simulink model "VehDyn14DOF"  (R2024b)
settings: Solver=VariableStepAuto  StartTime=0.0  StopTime=inf  FixedStep=0.001  RelTol=1e-3
model workspace (MAT data in the model file):
  ssEnable : Simulink.Parameter (value not decoded)
  xdot_r : Simulink.Parameter (value not decoded)
values from neighbouring files (symbols this model uses):
  AccPwrbp = 0.0 3.0779560993538198    [vehDyn14DOF.sldd]
  AccSpdbp = 256.49641719585139 641.24104298962845    [vehDyn14DOF.sldd]
  Downshift_Speeds = 9.5625 12.9375 16.3125 19.6875 23.0625 26.4375 29.8125 33.1875 36.5625 39.9375 43.3125 46.687499999999986 47.8125 51.187499999999986 54.562499999999986 57.9375 59.0625 62.4375 65.8125 69.1875 68.90625 72.84375 76.78125 80.71875 78.75 83.25 87.75 92.25    [vehDyn14DOF.sldd]
  egoVehDyn = egoVehicleDynamicsParamsFromRR(egoInitialPose, actorProfiles(egoActorID))    [helperSLTrajectoryFollowerWithRRScenarioSetup.m]
  EngRevLim = 7000.0    [vehDyn14DOF.sldd]
  F0z = 2886.0 2907.0    [vehDyn14DOF.sldd]
  Iz = evalin('base','Iz')    [helperSLTrajectoryFollowerWithRRScenarioSetup.m]
  lf = evalin('base','lf')    [helperSLTrajectoryFollowerWithRRScenarioSetup.m]
  lr = evalin('base','lr')    [helperSLTrajectoryFollowerWithRRScenarioSetup.m]
  m = worldActors(idx).actor_runtime.pose.matrix    [helperSLTrajectoryFollowerWithRRScenarioSetup.m]
  Pedal_Positions = 0.1 0.4 0.5 0.9    [vehDyn14DOF.sldd]
  steerGear = evalin('base', 'steerGear')    [helperSLTrajectoryFollowerWithRRScenarioSetup.m]
  steeringGain = evalin('base', 'steeringGain')    [helperSLTrajectoryFollowerWithRRScenarioSetup.m]
  steerLimit = evalin('base', 'steerLimit')    [helperSLTrajectoryFollowerWithRRScenarioSetup.m]
  Trans = 0.01    [vehDyn14DOF.sldd]
  Upshift_Speeds = 12.9375 16.3125 19.6875 33.0 26.4375 29.8125 33.1875 52.5 39.9375 43.3125 46.687499999999986 77.25 51.187499999999986 54.562499999999986 57.9375 100.5 62.4375 65.8125 69.1875 138.75 72.84375 76.78125 80.71875 161.875 83.25 87.75 92.25 185.0    [vehDyn14DOF.sldd]
  VEH = 1575.0    [vehDyn14DOF.sldd]
symbols that are objects in the model workspace (value not decoded): ssEnable, xdot_r
undefined symbols (not defined in the file or in its folder): AccelCmd, CurvGradRef, CurvRef, DecelCmd, DiscIntNeverNeededParam, EnblAccelCmd, EnblDecelCmd, EnblSteerCmd, GearCmd, Gnd, lambda_mux, lambda_muy, LngRef, LtrRef, max_ac, max_dc, PhiRef, SteerCmd, SteerZero, Wind, XRef, YRef, Z
libraries: simulink x14, autolibutils x13, autolibsharedcoupling x11, vehdynlibtire x10, vehdynlibsuspension x8, sharedtransform x5, autolibshareddiff x5, shared6dof x2, slpidlib x1, autolibtranscontrolscommon x1, vehdynlibdriver x1, autolibshared x1
(part 10 of 10)

== system VehDyn14DOF/Passenger Vehicle/Chassis and Tires/Wheels and Tires/VDBS/Tires/MF Tires/Fy ==
  In1 : Inport
  In2 : Inport  Port=2
  In3 : Inport  Port=3
  In4 : Inport  Port=4
  Bus Selector{,1..3} (4 alike) : BusSelector  OutputSignals=Fy
  Vector Concatenate : Concatenate  NumInputs=4
  Out1 : Outport  VectorParamsAs1DForOutWhenUnconnected=off
  wires:
  Vector Concatenate/1 -> Out1/1
  In1/1 -> Bus Selector/1
  Bus Selector/1 -> Vector Concatenate/1  "<Fy>"
  In2/1 -> Bus Selector1/1
  In3/1 -> Bus Selector2/1
  In4/1 -> Bus Selector3/1
  Bus Selector1/1 -> Vector Concatenate/2  "<Fy>"
  Bus Selector2/1 -> Vector Concatenate/3  "<Fy>"
  Bus Selector3/1 -> Vector Concatenate/4  "<Fy>"

== system VehDyn14DOF/Passenger Vehicle/Chassis and Tires/Wheels and Tires/VDBS/Tires/MF Tires/Fz ==
  In1 : Inport
  In2 : Inport  Port=2
  In3 : Inport  Port=3
  In4 : Inport  Port=4
  Bus Selector{,1..3} (4 alike) : BusSelector  OutputSignals=Fz
  Vector Concatenate : Concatenate  NumInputs=4
  Out1 : Outport  VectorParamsAs1DForOutWhenUnconnected=off
  wires:
  Vector Concatenate/1 -> Out1/1
  In1/1 -> Bus Selector/1
  Bus Selector/1 -> Vector Concatenate/1  "<Fz>"
  In2/1 -> Bus Selector1/1
  In3/1 -> Bus Selector2/1
  In4/1 -> Bus Selector3/1
  Bus Selector1/1 -> Vector Concatenate/2  "<Fz>"
  Bus Selector2/1 -> Vector Concatenate/3  "<Fz>"
  Bus Selector3/1 -> Vector Concatenate/4  "<Fz>"

== system VehDyn14DOF/Passenger Vehicle/Chassis and Tires/Wheels and Tires/VDBS/Tires/MF Tires/Mx ==
  In1 : Inport
  In2 : Inport  Port=2
  In3 : Inport  Port=3
  In4 : Inport  Port=4
  Bus Selector{,1..3} (4 alike) : BusSelector  OutputSignals=Mx
  Vector Concatenate : Concatenate  NumInputs=4
  Out1 : Outport  VectorParamsAs1DForOutWhenUnconnected=off
  wires:
  Vector Concatenate/1 -> Out1/1
  In1/1 -> Bus Selector/1
  Bus Selector/1 -> Vector Concatenate/1  "<Mx>"
  In2/1 -> Bus Selector1/1
  In3/1 -> Bus Selector2/1
  In4/1 -> Bus Selector3/1
  Bus Selector1/1 -> Vector Concatenate/2  "<Mx>"
  Bus Selector2/1 -> Vector Concatenate/3  "<Mx>"
  Bus Selector3/1 -> Vector Concatenate/4  "<Mx>"

== system VehDyn14DOF/Passenger Vehicle/Chassis and Tires/Wheels and Tires/VDBS/Tires/MF Tires/My ==
  In1 : Inport
  In2 : Inport  Port=2
  In3 : Inport  Port=3
  In4 : Inport  Port=4
  Bus Selector{,1..3} (4 alike) : BusSelector  OutputSignals=My
  Vector Concatenate : Concatenate  NumInputs=4
  Out1 : Outport  VectorParamsAs1DForOutWhenUnconnected=off
  wires:
  Bus Selector3/1 -> Vector Concatenate/4  "<My>"
  Bus Selector2/1 -> Vector Concatenate/3  "<My>"
  Bus Selector1/1 -> Vector Concatenate/2  "<My>"
  In4/1 -> Bus Selector3/1
  In3/1 -> Bus Selector2/1
  In2/1 -> Bus Selector1/1
  Bus Selector/1 -> Vector Concatenate/1  "<My>"
  In1/1 -> Bus Selector/1
  Vector Concatenate/1 -> Out1/1

== system VehDyn14DOF/Passenger Vehicle/Chassis and Tires/Wheels and Tires/VDBS/Tires/MF Tires/Mz ==
  In1 : Inport
  In2 : Inport  Port=2
  In3 : Inport  Port=3
  In4 : Inport  Port=4
  Bus Selector{,1..3} (4 alike) : BusSelector  OutputSignals=Mz
  Vector Concatenate : Concatenate  NumInputs=4
  Out1 : Outport  VectorParamsAs1DForOutWhenUnconnected=off
  wires:
  Bus Selector3/1 -> Vector Concatenate/4  "<Mz>"
  Bus Selector2/1 -> Vector Concatenate/3  "<Mz>"
  Bus Selector1/1 -> Vector Concatenate/2  "<Mz>"
  In4/1 -> Bus Selector3/1
  In3/1 -> Bus Selector2/1
  In2/1 -> Bus Selector1/1
  Bus Selector/1 -> Vector Concatenate/1  "<Mz>"
  In1/1 -> Bus Selector/1
  Vector Concatenate/1 -> Out1/1

== system VehDyn14DOF/Passenger Vehicle/Chassis and Tires/Wheels and Tires/VDBS/Tires/MF Tires/Re ==
  In1 : Inport
  In2 : Inport  Port=2
  In3 : Inport  Port=3
  In4 : Inport  Port=4
  Bus Selector{,1..3} (4 alike) : BusSelector  OutputSignals=Re
  Vector Concatenate : Concatenate  NumInputs=4
  Out1 : Outport  VectorParamsAs1DForOutWhenUnconnected=off
  wires:
  Vector Concatenate/1 -> Out1/1
  In1/1 -> Bus Selector/1
  Bus Selector/1 -> Vector Concatenate/1  "<Re>"
  In2/1 -> Bus Selector1/1
  In3/1 -> Bus Selector2/1
  In4/1 -> Bus Selector3/1
  Bus Selector1/1 -> Vector Concatenate/2  "<Re>"
  Bus Selector2/1 -> Vector Concatenate/3  "<Re>"
  Bus Selector3/1 -> Vector Concatenate/4  "<Re>"

== system VehDyn14DOF/Passenger Vehicle/Chassis and Tires/Wheels and Tires/VDBS/Tires/MF Tires/alpha ==
  In1 : Inport
  In2 : Inport  Port=2
  In3 : Inport  Port=3
  In4 : Inport  Port=4
  Bus Selector{,1..3} (4 alike) : BusSelector  OutputSignals=Alpha
  Vector Concatenate : Concatenate  NumInputs=4
  Out1 : Outport  VectorParamsAs1DForOutWhenUnconnected=off
  wires:
  Vector Concatenate/1 -> Out1/1
  In1/1 -> Bus Selector/1
  Bus Selector/1 -> Vector Concatenate/1  "<Alpha>"
  In2/1 -> Bus Selector1/1
  In3/1 -> Bus Selector2/1
  In4/1 -> Bus Selector3/1
  Bus Selector1/1 -> Vector Concatenate/2  "<Alpha>"
  Bus Selector2/1 -> Vector Concatenate/3  "<Alpha>"
  Bus Selector3/1 -> Vector Concatenate/4  "<Alpha>"

== system VehDyn14DOF/Passenger Vehicle/Chassis and Tires/Wheels and Tires/VDBS/Tires/MF Tires/kappa ==
  In1 : Inport
  In2 : Inport  Port=2
  In3 : Inport  Port=3
  In4 : Inport  Port=4
  Bus Selector{,1..3} (4 alike) : BusSelector  OutputSignals=Kappa
  Vector Concatenate : Concatenate  NumInputs=4
  Out1 : Outport  VectorParamsAs1DForOutWhenUnconnected=off
  wires:
  Bus Selector3/1 -> Vector Concatenate/4  "<Kappa>"
  Bus Selector2/1 -> Vector Concatenate/3  "<Kappa>"
  Bus Selector1/1 -> Vector Concatenate/2  "<Kappa>"
  In4/1 -> Bus Selector3/1
  In3/1 -> Bus Selector2/1
  In2/1 -> Bus Selector1/1
  Bus Selector/1 -> Vector Concatenate/1  "<Kappa>"
  In1/1 -> Bus Selector/1
  Vector Concatenate/1 -> Out1/1

== system VehDyn14DOF/Passenger Vehicle/Chassis and Tires/Wheels and Tires/VDBS/Tires/MF Tires/omega ==
  In1 : Inport
  In2 : Inport  Port=2
  In3 : Inport  Port=3
  In4 : Inport  Port=4
  Bus Selector{,1..3} (4 alike) : BusSelector  OutputSignals=Omega
  Vector Concatenate : Concatenate  NumInputs=4
  Out1 : Outport  VectorParamsAs1DForOutWhenUnconnected=off
  wires:
  In1/1 -> Bus Selector/1
  Bus Selector/1 -> Vector Concatenate/1  "<Omega>"
  In2/1 -> Bus Selector1/1
  In3/1 -> Bus Selector2/1
  In4/1 -> Bus Selector3/1
  Bus Selector1/1 -> Vector Concatenate/2  "<Omega>"
  Bus Selector2/1 -> Vector Concatenate/3  "<Omega>"
  Bus Selector3/1 -> Vector Concatenate/4  "<Omega>"
  Vector Concatenate/1 -> Out1/1

== system VehDyn14DOF/Passenger Vehicle/Chassis and Tires/Wheels and Tires/VDBS/Tires/MF Tires/z ==
  In1 : Inport
  In2 : Inport  Port=2
  In3 : Inport  Port=3
  In4 : Inport  Port=4
  Bus Selector{,1..3} (4 alike) : BusSelector  OutputSignals=z
  Vector Concatenate : Concatenate  NumInputs=4
  Out1 : Outport  VectorParamsAs1DForOutWhenUnconnected=off
  wires:
  Bus Selector3/1 -> Vector Concatenate/4  "<z>"
  Bus Selector2/1 -> Vector Concatenate/3  "<z>"
  Bus Selector1/1 -> Vector Concatenate/2  "<z>"
  In4/1 -> Bus Selector3/1
  In3/1 -> Bus Selector2/1
  In2/1 -> Bus Selector1/1
  Bus Selector/1 -> Vector Concatenate/1  "<z>"
  In1/1 -> Bus Selector/1
  Vector Concatenate/1 -> Out1/1

== system VehDyn14DOF/Passenger Vehicle/Chassis and Tires/Wheels and Tires/VDBS/Tires/MF Tires/zdot ==
  In1 : Inport
  In2 : Inport  Port=2
  In3 : Inport  Port=3
  In4 : Inport  Port=4
  Bus Selector{,1..3} (4 alike) : BusSelector  OutputSignals=zdot
  Vector Concatenate : Concatenate  NumInputs=4
  Out1 : Outport  VectorParamsAs1DForOutWhenUnconnected=off
  wires:
  Vector Concatenate/1 -> Out1/1
  In1/1 -> Bus Selector/1
  Bus Selector/1 -> Vector Concatenate/1  "<zdot>"
  In2/1 -> Bus Selector1/1
  In3/1 -> Bus Selector2/1
  In4/1 -> Bus Selector3/1
  Bus Selector1/1 -> Vector Concatenate/2  "<zdot>"
  Bus Selector2/1 -> Vector Concatenate/3  "<zdot>"
  Bus Selector3/1 -> Vector Concatenate/4  "<zdot>"

== stateflow chart VehDyn14DOF/Controllers/Transmission Controller/Transmission Controller/TCM/TCM Shift Controller ==
  settings: sampleTime=0.01
  state GearCmd [parallel]
    settings: executionOrder=1
    state Neutral
      en:
      GearCmd = 0;
    state G1
      en:
      GearCmd = 1;
    state G2
      en:
      GearCmd = 2;
      du:
      [SpdThr] = calc(2,pedal,speed);
    state G3
      en:
      GearCmd = 3;
      du:
      [SpdThr] = calc(3,pedal,speed);
    state G8
      en:
      GearCmd = 8;
    state G7
      en:
      GearCmd = 7;
    state G6
      en:
      GearCmd = 6;
    state G5
      en:GearCmd=5;
      du:[SpdThr]=calc(5,pedal,speed);
    state G4
      en:
      GearCmd = 4;
      du:
      [SpdThr] = calc(4,pedal,speed);
    (default) -> Neutral
    Neutral -> G1 : [~Neutral]
    G1 -> G2 [order 1] : Up
    G2 -> G3 [order 1] : Up
    G1 -> Neutral [order 2] : [Neutral]
    G2 -> G1 [order 2] : Down
    G3 -> G2 [order 2] : Down
    G3 -> G4 [order 1] : Up
    G4 -> G3 [order 2] : Down
    G7 -> G8 [order 1] : Up
    G5 -> G6 [order 1] : Up
    G6 -> G7 [order 1] : Up
    G4 -> G5 [order 1] : Up
    G5 -> G4 [order 2] : Down
    G6 -> G5 [order 2] : Down
    G7 -> G6 [order 2] : Down
    G8 -> G7 : Down
  state SelectionState [parallel]
    du:[up_th]=calc_up(GearCmd,pedal);
    du:[down_th]=calc_down(GearCmd,pedal);
    settings: executionOrder=2
    state SteadyState
      en:
      clutchControl = 0;
    state preDownShifting
    state preUpShifting
    state UpShifting
      en:
      GearCmd = GearCmd + 0.5;
    state DownShifting
      en:
      GearCmd = GearCmd - 0.5;
    (default) -> SteadyState
    SteadyState -> (junction 62) [order 1] : [speed < down_th && ...
        | GearCmd >1]
    SteadyState -> (junction 128) [order 2] : [speed > up_th &&...
        | GearCmd <= 5 && ...
        | floor(GearCmd) == GearCmd]
    (junction 62) -> preDownShifting
    (junction 128) -> preUpShifting
    (junction 168) -> SteadyState
    (junction 23) -> SteadyState
    (junction 161) -> SteadyState
    preDownShifting -> (junction 168) [order 2] : [speed >= down_th]
    preUpShifting -> (junction 161) [order 2] : [speed <= up_th]
    preUpShifting -> UpShifting [order 1] : after(0.5,sec)
        | [speed>up_th]
    preDownShifting -> DownShifting [order 1] : after(0.5, sec)
        | [speed < down_th - 2]
    DownShifting -> (junction 23) : {GearCmd.Down;}
    UpShifting -> (junction 23) : {GearCmd.Up;}
  state up_th = calc_up(gear,pedal) [function]
  state down_th = calc_down(gear,pedal) [function]
  state SpdThr = calc(gear,pedal,speed) [function]
  data: gear function_input; pedal function_input; up_th function_output; gear function_input; pedal function_input; down_th function_output; gear function_input; pedal function_input; SpdThr function_output; speed function_input; GearCmd output int8; speed input; pedal input; clutchControl local double; SpdThr local double; Neutral input; up_th local double; down_th local double
  events: Up local EITHER_EDGE_EVENT; Down local EITHER_EDGE_EVENT

== matlab function VehDyn14DOF/Passenger Vehicle/Chassis and Tires/Vehicle/Variant Subsystem/6DOF/Suspension to Chasiss Transforms/Estimated Unsprung Mass Orientation ==
  data: angles output size=3; angleIn input size=3; GeomXYZ output size=3; GemoXYZIn input size=3; Ground input size=4; trackW parameter; wheelB parameter
function [angles,GeomXYZ]= three26(angleIn, GemoXYZIn, Ground,trackW, wheelB)%#codegen
coder.allowpcode('plain')
% Copyright 2018 The MathWorks, Inc.
[angles,GeomXYZ]= vdynthree2six(angleIn, GemoXYZIn, Ground,trackW, wheelB);

== matlab function VehDyn14DOF/Controllers/Brake Pressure Control/Bang Bang ABS/Kappa/MATLAB Function ==
  data: Omega input; xdot input; KappaEst output
function KappaEst = fcn(Omega, xdot)

Re = 0.29;
KappaEst = 0;
WhlSpd = Omega * Re;

if xdot*WhlSpd ~= 0
    KappaEst = (WhlSpd - xdot)/max([abs(xdot) abs(WhlSpd)]);
end

== matlab function VehDyn14DOF/Controllers/Brake Pressure Control/Five-State ABS/Wheel Accel and Slip Estimator/Kappa/MATLAB Function ==
  data: Omega input; xdot input; KappaEst output
function KappaEst = fcn(Omega, xdot)

Re = 0.29;
KappaEst = 0;
WhlSpd = Omega * Re;

if xdot*WhlSpd ~= 0
    KappaEst = (WhlSpd - xdot)/max([abs(xdot) abs(WhlSpd)]);
end

== stateflow chart VehDyn14DOF/Controllers/Brake Pressure Control/Five-State ABS/ABSCtrlForEach/For Each Subsystem/ABSForEachWheel ==
  state ABSOff
    entry:
    PbOutput = Pref_dot;
    Flag = 0;
    during:
    PbOutput = Pref_dot;
  state Normal
    entry:
    PbOutput = Pref_dot;
    Flag = 0;
    during:
    PbOutput = Pref_dot;
  state ABSOn
    state Phase1
      entry:
      PbOutput = v1;
      Flag = 1;
    state Phase5
      entry:
      PbOutput = v5;
      Flag = 5;
    state Phase2
      entry:
      PbOutput = 0;
      Flag = 2;
    state Phase4
      entry:
      PbOutput = 0;
      Flag = 4;
    state Phase3
      entry:
      PbOutput = v4;
      Flag = 3;
    (default) -> Phase1
    Phase5 -> Phase1 : [e2 < a2]
    Phase1 -> Phase2 : [e2 >= b]
    Phase4 -> Phase5 : [e2 <= a1]
    Phase2 -> Phase3 : [e2 >= A]
    Phase3 -> Phase4 : [e2 < A]
  (default) -> ABSOff
  ABSOn -> ABSOff : [abs(VehSpd) < 2 || Pref <= 0]
  Normal -> ABSOff [order 2] : [Pref <= 0]
  ABSOff -> Normal : [Pref > 0 && e2 < a2]
  Normal -> ABSOn [order 1] : [e1 < 0]
  data: e1 input; e2 input; PbOutput output; Flag output; b parameter; v1 parameter; v4 parameter; v5 parameter; A parameter; a2 parameter; a1 parameter; Pref_dot input; Pref input; VehSpd input
